simulink library "lib_Convection_CylCrossFlowZukauskas"  (R2015a)
settings: Solver=ode45  StartTime=0.0  StopTime=10.0  RelTol=1e-3
libraries: simulink x10, lib_GenTools_MinMax x1
settings Model: Creator=jlkratz  LastModifiedBy=jlkratz

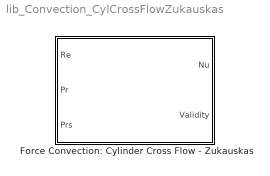
== system lib_Convection_CylCrossFlowZukauskas ==
  Force Convection: Cylinder Cross Flow - Zukauskas : Subsystem  mask(TSAT: Cylinder Cross Flow - Zukauskas){}
      mask help:
      | This block estimates the average Nusselt number of an external flow over an isothermal cylinder. The correlation employed was developed by Zukauskas and is a modification to an equation developed by Hilpert in order to better account for property variations. The Reynolds number (Re) should be calculated based on the cylinder diameter. All properties of the fluid except Prs, the Prandtl number calculated at the surface temperature, should be evaluated at the free stream temperature (NOT FILM TEMPERATURE LIKE THE HILPERT EQUATION). The correlation is subject to the following restrictions:
      |
      | 1 <= Re <= 1000000
      | 0.7 <= Pr <= 500
      |
      | Pr is the Prandtl number. For more information see the block help menu.
      mask Help: web(which('Convection_TSAT_CylinderCrossFlowZukauskas.html'),'-helpbrowser')

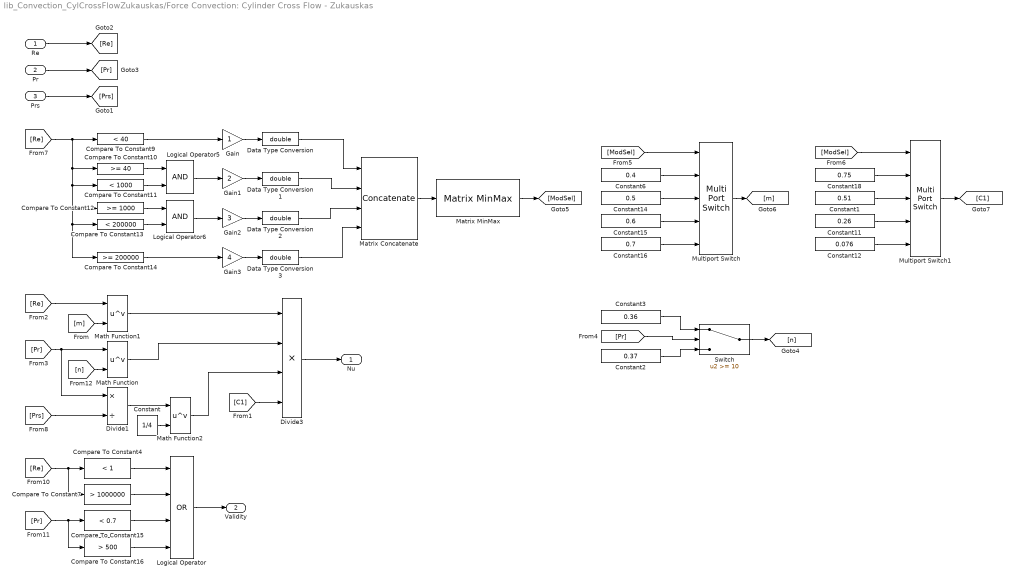
== system lib_Convection_CylCrossFlowZukauskas/Force Convection: Cylinder Cross Flow - Zukauskas ==
  Re : Inport
  Pr : Inport  Port=2
  Prs : Inport  Port=3
  Compare To Constant10 : simulink/Logic and Bit Operations/Compare To Constant  relop=>=  const=40  OutDataTypeStr=boolean
  Compare To Constant11 : simulink/Logic and Bit Operations/Compare To Constant  relop=<  const=1000  OutDataTypeStr=boolean
  Compare To Constant12 : simulink/Logic and Bit Operations/Compare To Constant  relop=>=  const=1000  OutDataTypeStr=boolean
  Compare To Constant13 : simulink/Logic and Bit Operations/Compare To Constant  relop=<  const=200000  OutDataTypeStr=boolean
  Compare To Constant14 : simulink/Logic and Bit Operations/Compare To Constant  relop=>=  const=200000  OutDataTypeStr=boolean
  Compare To Constant15 : simulink/Logic and Bit Operations/Compare To Constant  relop=<  const=0.7  OutDataTypeStr=boolean
  Compare To Constant16 : simulink/Logic and Bit Operations/Compare To Constant  relop=>  const=500  OutDataTypeStr=boolean
  Compare To Constant4 : simulink/Logic and Bit Operations/Compare To Constant  relop=<  const=1  OutDataTypeStr=boolean
  Compare To Constant7 : simulink/Logic and Bit Operations/Compare To Constant  relop=>  const=1000000  OutDataTypeStr=boolean
  Compare To Constant9 : simulink/Logic and Bit Operations/Compare To Constant  relop=<  const=40  OutDataTypeStr=boolean
  Constant : Constant  Value=1/4
  Constant1 : Constant  Value=0.51
  Constant11 : Constant  Value=0.26
  Constant12 : Constant  Value=0.076
  Constant14 : Constant  Value=0.5
  Constant15 : Constant  Value=0.6
  Constant16 : Constant  Value=0.7
  Constant18 : Constant  Value=0.75
  Constant2 : Constant  Value=0.37
  Constant3 : Constant  Value=0.36
  Constant6 : Constant  Value=0.4
  Data Type Conversion{,1..3} (4 alike) : DataTypeConversion  OutDataTypeStr=double
  Divide1 : Product  Inputs=*/
  Divide3 : Product  Inputs=****
  Gain : Gain
  Gain1 : Gain  Gain=2
  Gain2 : Gain  Gain=3
  Gain3 : Gain  Gain=4
  Logical Operator : Logic  Operator=OR  Inputs=4  AllPortsSameDT=off  OutDataTypeStr=boolean
  Logical Operator5 : Logic  AllPortsSameDT=off  OutDataTypeStr=boolean
  Logical Operator6 : Logic  AllPortsSameDT=off  OutDataTypeStr=boolean
  Math Function : Math  Operator=pow  SaturateOnIntegerOverflow=on
  Math Function1 : Math  Operator=pow  SaturateOnIntegerOverflow=on
  Math Function2 : Math  Operator=pow  SaturateOnIntegerOverflow=on
  Matrix Concatenate : Concatenate  NumInputs=4  Mode=Multidimensional array  ConcatenateDimension=2
  Matrix MinMax : lib_GenTools_MinMax/Matrix MinMax  rows_M=on  cols_M=off  all_M=off  minmax_M=off  BN_M=gcb
  Multiport Switch : MultiPortSwitch  Inputs=4
  Multiport Switch1 : MultiPortSwitch  Inputs=4
  Switch : Switch  Threshold=10
  Nu : Outport
  Validity : Outport  Port=2
  wires:
  Compare To Constant16/1 -> Logical Operator/4
  Compare To Constant15/1 -> Logical Operator/3
  Compare To Constant7/1 -> Logical Operator/2
  Compare To Constant4/1 -> Logical Operator/1
  [Pr] -> Compare To Constant15/1, Compare To Constant16/1
  [Re] -> Compare To Constant4/1, Compare To Constant7/1
  Math Function2/1 -> Divide3/3
  Math Function/1 -> Divide3/2
  Math Function1/1 -> Divide3/1
  [C1] -> Divide3/4
  Constant/1 -> Math Function2/2
  Divide1/1 -> Math Function2/1
  [Prs] -> Divide1/2
  [Pr] -> Math Function/1, Divide1/1
  [Re] -> Math Function1/1
  Prs/1 -> [Prs]
  Compare To Constant14/1 -> Gain3/1
  Compare To Constant9/1 -> Gain/1
  Logical Operator5/1 -> Gain1/1
  Logical Operator6/1 -> Gain2/1
  Compare To Constant12/1 -> Logical Operator6/1
  Compare To Constant13/1 -> Logical Operator6/2
  Compare To Constant10/1 -> Logical Operator5/1
  Compare To Constant11/1 -> Logical Operator5/2
  [Re] -> Compare To Constant12/1, Compare To Constant13/1, Compare To Constant14/1, Compare To Constant11/1, Compare To Constant10/1, Compare To Constant9/1
  Matrix Concatenate/1 -> Matrix MinMax/1
  Data Type Conversion3/1 -> Matrix Concatenate/4
  Data Type Conversion2/1 -> Matrix Concatenate/3
  Data Type Conversion1/1 -> Matrix Concatenate/2
  Data Type Conversion/1 -> Matrix Concatenate/1
  Matrix MinMax/1 -> [ModSel]
  Constant12/1 -> Multiport Switch1/5
  Constant11/1 -> Multiport Switch1/4
  Constant1/1 -> Multiport Switch1/3
  Constant18/1 -> Multiport Switch1/2
  Constant16/1 -> Multiport Switch/5
  Constant15/1 -> Multiport Switch/4
  Constant14/1 -> Multiport Switch/3
  Constant6/1 -> Multiport Switch/2
  Multiport Switch1/1 -> [C1]
  Multiport Switch/1 -> [m]
  [ModSel] -> Multiport Switch1/1
  [ModSel] -> Multiport Switch/1
  Gain3/1 -> Data Type Conversion3/1
  Gain2/1 -> Data Type Conversion2/1
  Gain1/1 -> Data Type Conversion1/1
  Gain/1 -> Data Type Conversion/1
  Pr/1 -> [Pr]
  Re/1 -> [Re]
  Logical Operator/1 -> Validity/1
  Divide3/1 -> Nu/1
  [m] -> Math Function1/2
  [n] -> Math Function/2
  [Pr] -> Switch/2
  Constant3/1 -> Switch/1
  Constant2/1 -> Switch/3
  Switch/1 -> [n]
